simulink model "deadReckoningPlant"  (R2017a)
settings: Solver=FixedStepDiscrete  StartTime=0.0  StopTime=10  FixedStep=0.01  RelTol=1e-3
PreLoadFcn:
  | robotParameters;
values from neighbouring files (symbols this model uses):
  ticksPerRot = 627.2    [robotParameters.m]
  wheelR = 0.052    [robotParameters.m]
undefined symbols (not defined in the file or in its folder): motorIp, motorSp
libraries: mobileRoboticsTrainingLib x5
settings Model: Creator=sseshadr  LastModifiedBy=shiremat

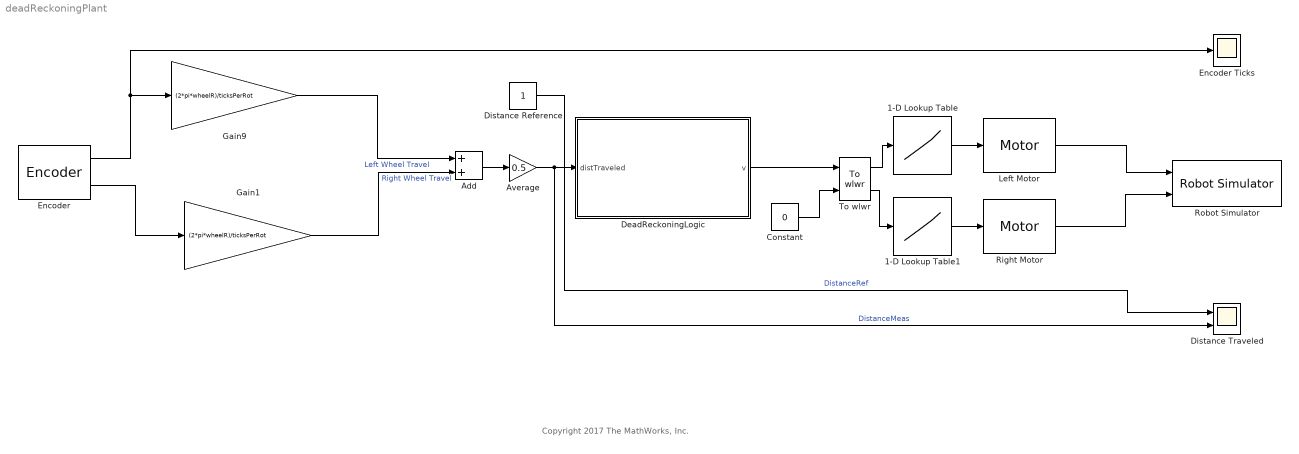
== system deadReckoningPlant ==
  note: Copyright 2017 The MathWorks, Inc.
  1-D Lookup Table : Lookup_n-D  NumberOfTableDimensions=1  BreakpointsForDimension1=motorSp  Table=motorIp  ExtrapMethod=Clip  InternalRulePriority=Speed  RndMeth=Simplest  InputSameDT=on
  1-D Lookup Table1 : Lookup_n-D  NumberOfTableDimensions=1  BreakpointsForDimension1=motorSp  Table=motorIp  ExtrapMethod=Clip  InternalRulePriority=Speed  RndMeth=Simplest  InputSameDT=on
  Add : Sum
  Average : Gain  Gain=0.5
  Constant : Constant  Value=0
  DeadReckoningLogic : Stateflow chart  TreatAsAtomicUnit=on
  Distance Reference : Constant
  Distance Traveled : Scope  NumInputPorts=2
  Encoder : mobileRoboticsTrainingLib/Encoder  axleLength=axleLength  wheelR=wheelR  ticksPerRot=ticksPerRot
      settings: SourceProductName=Mobile Robotics Training Library
  Encoder Ticks : Scope
  Gain1 : Gain  Gain=(2*pi*wheelR)/ticksPerRot
  Gain9 : Gain  Gain=(2*pi*wheelR)/ticksPerRot
  Left Motor : mobileRoboticsTrainingLib/Motor  motorPlant=wheelMotorModel  sensorType=Speed
      settings: SourceProductName=Mobile Robotics Training Library
  Right Motor : mobileRoboticsTrainingLib/Motor  motorPlant=wheelMotorModel  sensorType=Speed
      settings: SourceProductName=Mobile Robotics Training Library
  Robot Simulator : mobileRoboticsTrainingLib/Robot Simulator  Priority=99  mapVar=[]  startX=2  startY=2  startTheta=0  axleLength=axleLength  wheelR=wheelR
  To wlwr : mobileRoboticsTrainingLib/To wlwr  axleLength=0.1  wheelR=0.05
  wires:
  Average/1 -> Distance Traveled/2, DeadReckoningLogic/1(distTraveled)  "DistanceMeas"
  Gain9/1 -> Add/1  "Left Wheel Travel"
  Add/1 -> Average/1
  Gain1/1 -> Add/2  "Right Wheel Travel"
  Encoder/1 -> Gain9/1, Encoder Ticks/1
  Encoder/2 -> Gain1/1
  Constant/1 -> To wlwr/2
  DeadReckoningLogic/1(v) -> To wlwr/1
  To wlwr/1 -> 1-D Lookup Table/1
  1-D Lookup Table/1 -> Left Motor/1
  1-D Lookup Table1/1 -> Right Motor/1
  Left Motor/1 -> Robot Simulator/1
  To wlwr/2 -> 1-D Lookup Table1/1
  Right Motor/1 -> Robot Simulator/2
  Distance Reference/1 -> Distance Traveled/1  "DistanceRef"

== stateflow chart deadReckoningPlant/DeadReckoningLogic ==
  state MoveForward
    entry:
    v = 0.5;
  state Stop
    entry:
    v = 0;
  (default) -> MoveForward : %Start Dead Reckoning
  MoveForward -> Stop : [distTraveled >= 1]
  data: v output; distTraveled input
